simulink model "model_cuk"  (R2022b)
settings: Solver=ode45  StartTime=0.0  StopTime=0.05  RelTol=1e-3  EnableMultiTasking=on
values from neighbouring files (symbols this model uses):
  C = 22e-6    (= 2.2e-05)    [loop_buck_boost.m]    (also in loop_cuk.m; var_buck_boost.m; var_cuk.m)
  C1 = 1e-6    (= 1e-06)    [loop_cuk.m]    (also in var_cuk.m)
  fD = 50    [loop_cuk.m]    (also in var_cuk.m)
  fL = 100    [loop_cuk.m]    (also in var_cuk.m)
  L = 1e-3    (= 0.001)    [loop_buck_boost.m]    (also in loop_cuk.m = 4.7e-05; var_buck_boost.m; var_cuk.m = 4.7e-05)
  L1 = 15e-6    (= 1.5e-05)    [loop_cuk.m]    (also in var_cuk.m)
  LL = 5e-3    (= 0.005)    [loop_buck_boost.m]    (also in loop_cuk.m = 0.001; sim_buck_boost.m = LLs(i); sim_cuk.m = LLs(i); var_buck_boost.m)
  rC = 10e-3    (= 0.01)    [loop_cuk.m]    (also in var_cuk.m)
  rC1 = 10e-3    (= 0.01)    [loop_cuk.m]    (also in var_cuk.m)
  rL = 20e-3    (= 0.02)    [loop_buck_boost.m]    (also in loop_cuk.m = 0.03; var_buck_boost.m; var_cuk.m = 0.03)
  rL1 = 35e-3    (= 0.035)    [loop_cuk.m]    (also in var_cuk.m)
  RL_med = 20    [loop_cuk.m]    (also in var_cuk.m)
  rs = 25e-3    (= 0.025)    [loop_buck_boost.m]    (also in loop_cuk.m = 0.03; var_buck_boost.m; var_cuk.m = 0.03)
  Vd = 10    [loop_cuk.m]    (also in var_cuk.m)
settings Model: Creator=11802972  LastModifiedBy=andre
settings SolverCC: AlgebraicLoopSolver=TrustRegion
settings DataIOCC: LimitDataPoints=on  SaveFormat=Array  ReturnWorkspaceOutputs=off
settings OptimizationCC: LifeSpan=inf
settings DebuggingCC: UnconnectedInputMsg=warning  UnconnectedOutputMsg=warning  UnconnectedLineMsg=warning  SFUnexpectedBacktrackingDiag=warning  SFNoUnconditionalDefaultTransitionDiag=warning  SFExecutionAtInitializationDiag=none  SFMachineParentedDataDiag=warning  ArithmeticOperatorsInVariantConditions=warning
settings HardwareCC: ProdBitPerPointer=32  ProdBitPerSizeT=32  ProdBitPerPtrDiffT=32  ProdLargestAtomicFloat=None  ProdIntDivRoundTo=Undefined  ProdEndianess=Unspecified  ProdWordSize=32  ProdHWDeviceType=32-bit Generic
settings ModelReferenceCC: PropagateSignalLabelsOutOfModel=off
settings SFSimCC: SimUseLocalCustomCode=off  CustomCodeUndefinedFunction=UseInterfaceOnly
settings RTWCC: RTWUseLocalCustomCode=off
settings CodeAppCC: StateflowObjectComments=on
settings GRTTargetCC: TargetLangStandard=C89/C90 (ANSI)
settings ConfigComp: CovMetricSettings=dw  CovSaveCumulativeToWorkspaceVar=on  CovSaveSingleToWorkspaceVar=on  CovExternalEMLEnable=off

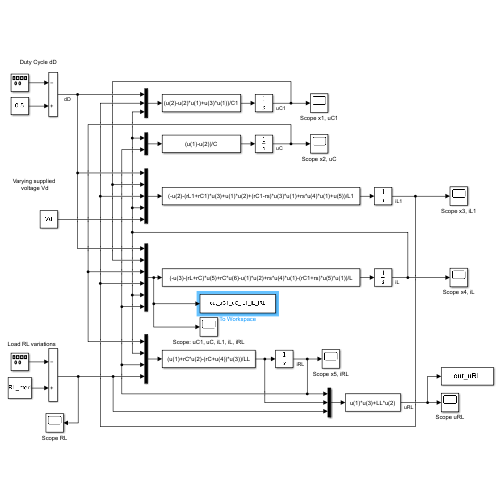
[thumbnail: Simulink's stored preview of the top-level diagram]
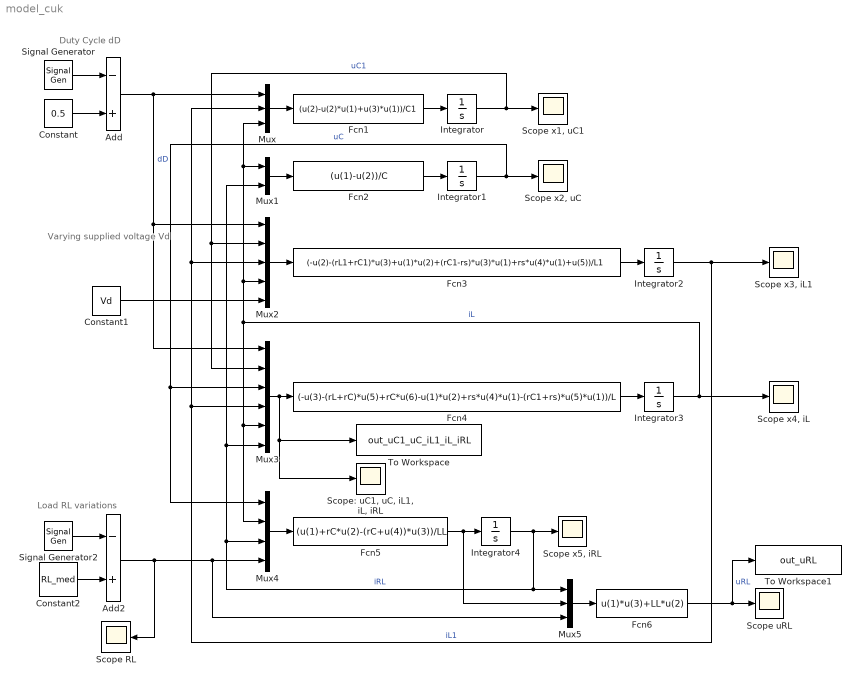
== system model_cuk ==
  note: Duty Cycle dD
  note: Varying supplied
      | voltage Vd
  note: Load RL variations
  Add : Sum  Inputs=-+
  Add2 : Sum  Inputs=-+
  Constant : Constant  Value=0.5
  Constant1 : Constant  Value=Vd
  Constant2 : Constant  Value=RL_med
  Fcn1 : Fcn  Expr=(u(2)-u(2)*u(1)+u(3)*u(1))/C1
  Fcn2 : Fcn  Expr=(u(1)-u(2))/C
  Fcn3 : Fcn  Expr=(-u(2)-(rL1+rC1)*u(3)+u(1)*u(2)+(rC1-rs)*u(3)*u(1)+rs*u(4)*u(1)+u(5))/L1
  Fcn4 : Fcn  Expr=(-u(3)-(rL+rC)*u(5)+rC*u(6)-u(1)*u(2)+rs*u(4)*u(1)-(rC1+rs)*u(5)*u(1))/L
  Fcn5 : Fcn  Expr=(u(1)+rC*u(2)-(rC+u(4))*u(3))/LL
  Fcn6 : Fcn  Expr=u(1)*u(3)+LL*u(2)
  Integrator{,1..4} (5 alike) : Integrator
  Mux : Mux  Inputs=3
  Mux1 : Mux  Inputs=2
  Mux2 : Mux  Inputs=5
  Mux3 : Mux  Inputs=6
  Mux4 : Mux
  Mux5 : Mux  Inputs=3
  Scope RL : Scope
  Scope uRL : Scope
  "Scope x1, uC1" : Scope
  "Scope x2, uC" : Scope
  "Scope x3, iL1" : Scope
  "Scope x4, iL" : Scope
  "Scope x5, iRL" : Scope
  "Scope: uC1, uC, iL1, iL, iRL" : Scope
  Signal Generator : SignalGenerator  WaveForm=square  Amplitude=0.25  Frequency=fD
  Signal Generator2 : SignalGenerator  WaveForm=square  Amplitude=10  Frequency=fL
  To Workspace : ToWorkspace  VariableName=out_uC1_uC_iL1_iL_iRL  SaveFormat=Timeseries  SampleTime=-1
  To Workspace1 : ToWorkspace  VariableName=out_uRL  SaveFormat=Timeseries  SampleTime=-1
  wires:
  Signal Generator/1 -> Add/1
  Constant/1 -> Add/2
  Constant2/1 -> Add2/2
  Signal Generator2/1 -> Add2/1
  Add/1 -> Mux3/1, Mux2/1, Mux/1  "dD"
  Mux/1 -> Fcn1/1
  Fcn1/1 -> Integrator/1
  Mux1/1 -> Fcn2/1
  Fcn2/1 -> Integrator1/1
  Integrator/1 -> Mux3/2, Mux2/2, "Scope x1, uC1"/1  "uC1"
  Integrator1/1 -> Mux4/1, Mux3/3, "Scope x2, uC"/1  "uC"
  Mux2/1 -> Fcn3/1
  Fcn3/1 -> Integrator2/1
  Integrator2/1 -> Mux2/3, Mux/2, Mux3/4, "Scope x3, iL1"/1  "iL1"
  Mux3/1 -> "Scope: uC1, uC, iL1, iL, iRL"/1, To Workspace/1, Fcn4/1
  Integrator3/1 -> Mux2/4, Mux1/1, Mux/3, Mux4/2, Mux3/5, "Scope x4, iL"/1  "iL"
  Fcn4/1 -> Integrator3/1
  Mux4/1 -> Fcn5/1
  Fcn5/1 -> Mux5/2, Integrator4/1
  Integrator4/1 -> Mux5/1, Mux1/2, Mux3/6, Mux4/3, "Scope x5, iRL"/1  "iRL"
  Mux5/1 -> Fcn6/1
  Fcn6/1 -> To Workspace1/1, Scope uRL/1  "uRL"
  Constant1/1 -> Mux2/5
  Add2/1 -> Scope RL/1, Mux5/3, Mux4/4
